simulink model "Deployment_Dispositivo_Gruppo8"  (R2022b)
settings: Solver=FixedStepAuto  StartTime=0.0  StopTime=inf  FixedStep=0.01  RelTol=1e-3  EnableMultiTasking=on
libraries: mbedblockslib x7
settings Model: PacingRate=0.500000  ExtModeTrigDuration=10  Creator=kiraa  LastModifiedBy=kiraa
settings OptimizationCC: EnhancedBackFolding=on  PassReuseOutputArgsAs=Individual arguments  ZeroExternalMemoryAtStartup=off  ZeroInternalMemoryAtStartup=off  MaxStackSize=64  OptimizeBlockOrder=speed  DifferentSizesBufferReuse=on  OptimizationCustomize=off  EfficientTunableParamExpr=on
settings DebuggingCC: ParameterTunabilityLossMsg=error
settings HardwareCC: ProdBitPerPointer=32  ProdBitPerSizeT=32  ProdBitPerPtrDiffT=32  ProdLargestAtomicInteger=Long  ProdLargestAtomicFloat=Double  ProdWordSize=32  ProdLongLongMode=on  ProdHWDeviceType=ARM Compatible->ARM Cortex  UseEmbeddedCoderFeatures=off
settings SFSimCC: MATLABDynamicMemAlloc=off
settings RTWCC: Description=Embedded Coder  SystemTargetFile=ert.tlc  HardwareBoard=STM32 Nucleo F401RE  TLCOptions=-aInlineSetEventsForThisBaseRateFcn=TLC_FALSE -aSuppressMultiTaskScheduler=TLC_FALSE -aRateBasedStepFcn=1  TemplateMakefile=ert_default_tmf  Toolchain=GNU Tools for ARM Embedded Processors
settings CodeAppCC: ForceParamTrailComments=on  IgnoreCustomStorageClasses=off  OperatorAnnotations=on  SimulinkDataObjDesc=on  SFDataObjDesc=on  InsertBlockDesc=on
settings ERTTargetCC: SupportNonInlinedSFcns=on  ExtModeTransport=3  ExtModeStaticAlloc=on  ExtModeStaticAllocSize=2000  ExtModeMexFile=ext_xcp  ExtModeIntrfLevel=Level2 - Open

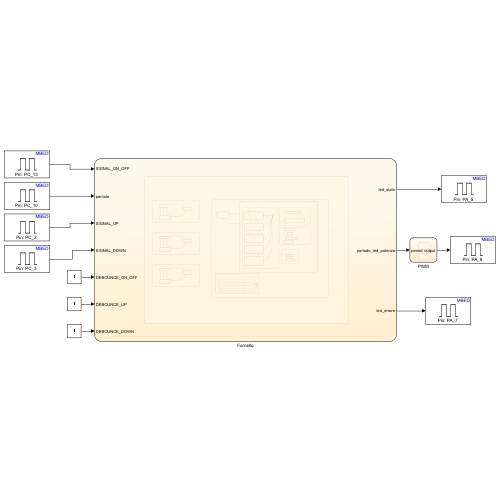
[thumbnail: Simulink's stored preview of the top-level diagram]
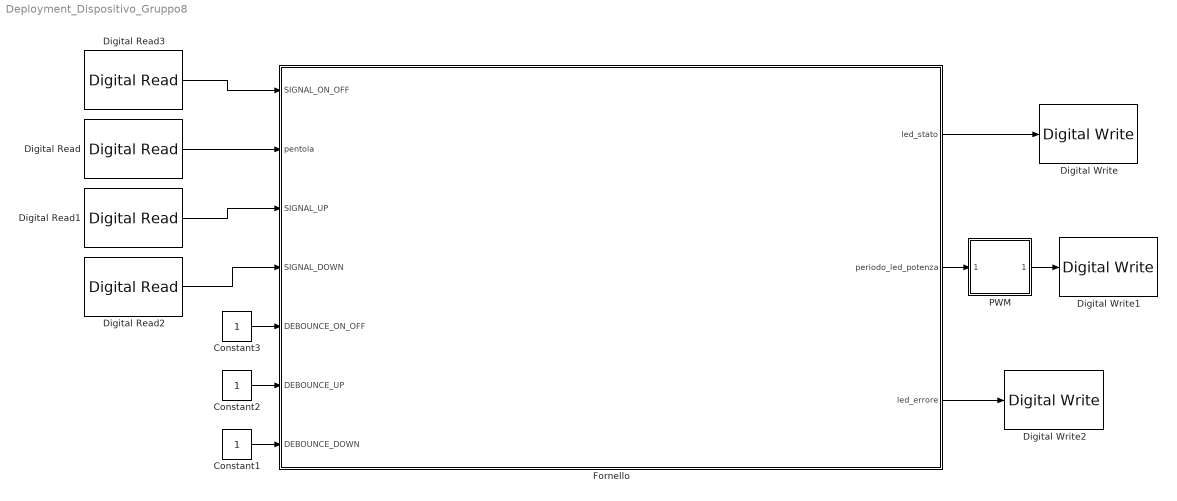
== system Deployment_Dispositivo_Gruppo8 ==
  Constant1 : Constant
  Constant2 : Constant
  Constant3 : Constant
  Digital Read : mbedblockslib/Digital Read  Pin=PC_10  Direction=input  SampleTime=-1
      settings: LibrarySourceBlock=stmnucleorootlib/Common/Digital Read
  Digital Read1 : mbedblockslib/Digital Read  Pin=PC_2  Direction=input  SampleTime=-1
      settings: LibrarySourceBlock=stmnucleorootlib/Common/Digital Read
  Digital Read2 : mbedblockslib/Digital Read  Pin=PC_3  Direction=input  SampleTime=-1
      settings: LibrarySourceBlock=stmnucleorootlib/Common/Digital Read
  Digital Read3 : mbedblockslib/Digital Read  Pin=PC_13  Direction=input  SampleTime=-1
      settings: LibrarySourceBlock=stmnucleorootlib/Common/Digital Read
  Digital Write : mbedblockslib/Digital Write  Pin=PA_5  Direction=output
      settings: LibrarySourceBlock=stmnucleorootlib/Common/Digital Write
  Digital Write1 : mbedblockslib/Digital Write  Pin=PA_6  Direction=output
      settings: LibrarySourceBlock=stmnucleorootlib/Common/Digital Write
  Digital Write2 : mbedblockslib/Digital Write  Pin=PA_7  Direction=output
      settings: LibrarySourceBlock=stmnucleorootlib/Common/Digital Write
  Fornello : Stateflow chart  TreatAsAtomicUnit=on
  PWM : Stateflow chart  TreatAsAtomicUnit=on
  wires:
  Fornello/1(led_stato) -> Digital Write/1
  Fornello/3(led_errore) -> Digital Write2/1
  Fornello/2(periodo_led_potenza) -> PWM/1(period)
  PWM/1(output) -> Digital Write1/1
  Constant1/1 -> Fornello/7(DEBOUNCE_DOWN)
  Constant2/1 -> Fornello/6(DEBOUNCE_UP)
  Constant3/1 -> Fornello/5(DEBOUNCE_ON_OFF)
  Digital Read1/1 -> Fornello/3(SIGNAL_UP)
  Digital Read/1 -> Fornello/2(pentola)
  Digital Read2/1 -> Fornello/4(SIGNAL_DOWN)
  Digital Read3/1 -> Fornello/1(SIGNAL_ON_OFF)

== stateflow chart Deployment_Dispositivo_Gruppo8/Fornello ==
  settings: executeAtInitialization=1
  state DEVICE
    state FORNELLO [parallel]
      settings: executionOrder=1
      state ON
        en: led_stato = true
        state SELECTOR [parallel]
          settings: executionOrder=1
          state SELECTED_0W
            en: selected_power=0;
          state SELECTED_300W
            en: selected_power=300;
          state SELECTED_500W
            en: selected_power=500
          state SELECTED_1000W
            en: selected_power=1000
          state SELECTED_1500W
            en: selected_power=1500
          (default) -> SELECTED_0W
          (junction 32) -> SELECTED_0W
          SELECTED_500W -> (junction 32) [order 1] : disattiva
          SELECTED_1000W -> (junction 32) [order 2] : disattiva
          SELECTED_1500W -> (junction 32) [order 2] : disattiva
          SELECTED_300W -> (junction 32) [order 1] : disattiva
          SELECTED_0W -> SELECTED_300W : LONG_PRESS_UP[pentola == false]
          SELECTED_300W -> SELECTED_0W [order 3] : LONG_PRESS_DOWN[pentola==false]
          SELECTED_500W -> SELECTED_300W [order 2] : LONG_PRESS_DOWN[pentola==false]
          SELECTED_300W -> SELECTED_500W [order 2] : LONG_PRESS_UP[pentola == false]
          SELECTED_1000W -> SELECTED_500W [order 3] : LONG_PRESS_DOWN[pentola==false]
          SELECTED_500W -> SELECTED_1000W [order 3] : LONG_PRESS_UP[pentola == false]
          SELECTED_1500W -> SELECTED_1000W [order 1] : LONG_PRESS_DOWN[pentola == false]
          SELECTED_1000W -> SELECTED_1500W [order 1] : LONG_PRESS_UP[pentola==false]
        state WATCHDOG [parallel]
          settings: executionOrder=2
          state IDLE
          state ERROR
            en: led_errore = true
            on after(10,sec): send(disattiva,SELECTOR); erogaPotenza(0)
            ex: led_errore = false
          (default) -> DEVICE.FORNELLO.ON.WATCHDOG.IDLE
          DEVICE.FORNELLO.ON.WATCHDOG.IDLE -> ERROR : [pentola == true && attivo==true]
          ERROR -> DEVICE.FORNELLO.ON.WATCHDOG.IDLE : [pentola == false || attivo == false]
        state SUPPLIER [parallel]
          settings: executionOrder=3
          state NO_CHANGE_REQUESTED
          state Applying_0_power
            en: erogaPotenza(selected_power)
          state Applying_power
            en: erogaPotenza(selected_power)
          state PENDING_CHANGE
            en: t_debug = 0
          NO_CHANGE_REQUESTED -> PENDING_CHANGE : change_power
          Applying_power -> NO_CHANGE_REQUESTED [order 2]
          Applying_0_power -> NO_CHANGE_REQUESTED
          Applying_power -> Applying_0_power [order 1] : [attivo == false]
          PENDING_CHANGE -> Applying_power : [pentola==false]
        state DELAYED_TRIGGER [parallel]
          settings: executionOrder=4
          state IDLE
          state DELAYING
          (default) -> DEVICE.FORNELLO.ON.DELAYED_TRIGGER.IDLE
          DEVICE.FORNELLO.ON.DELAYED_TRIGGER.IDLE -> DELAYING : change(selected_power)
          DELAYING -> DEVICE.FORNELLO.ON.DELAYED_TRIGGER.IDLE [order 2] : after(5,sec)/{send(change_power, SUPPLIER)}
          DELAYING -> DELAYING [order 1] : change(selected_power)
        (default) -> NO_CHANGE_REQUESTED
      state OFF
        en: led_stato = false; erogaPotenza(0)
      state erogaPotenza(power) [function]
        (default) -> (junction 65) : {power = double(power)}
        (junction 65) -> (junction 68) [order 1] : [power == 0]
        (junction 68) -> (junction 118) : {periodo_led_potenza=0;attivo=false}
        (junction 118) -> (junction 89)
        (junction 65) -> (junction 77) [order 2]
        (junction 77) -> (junction 83) [order 1] : [power == 300]
        (junction 83) -> (junction 120) : {periodo_led_potenza=2;attivo=true}
        (junction 120) -> (junction 89)
        (junction 77) -> (junction 79) [order 2]
        (junction 122) -> (junction 89)
        (junction 119) -> (junction 89)
        (junction 121) -> (junction 89)
        (junction 79) -> (junction 84) [order 1] : [power == 500]
        (junction 84) -> (junction 122) : {periodo_led_potenza=1;attivo=true}
        (junction 79) -> (junction 81) [order 2]
        (junction 81) -> (junction 92) [order 1] : [power == 1000]
        (junction 92) -> (junction 119) : {periodo_led_potenza=0.5;attivo=true}
        (junction 81) -> (junction 95) [order 2]
        (junction 95) -> (junction 99) : [power == 1500]
        (junction 99) -> (junction 121) : {periodo_led_potenza=0.25;attivo=true}
      (default) -> OFF
      OFF -> ON : SHORT_PRESS_ON_OFF
      ON -> OFF : LONG_PRESS_ON_OFF
    state BUTTON_ON_OFF [parallel]
      settings: executionOrder=2
      state HIGH
      state LOW_2
      state LOW
      (default) -> DEVICE.BUTTON_ON_OFF.HIGH
      DEVICE.BUTTON_ON_OFF.LOW_2 -> DEVICE.BUTTON_ON_OFF.HIGH : [SIGNAL_ON_OFF == true]
      DEVICE.BUTTON_ON_OFF.HIGH -> DEVICE.BUTTON_ON_OFF.LOW : [SIGNAL_ON_OFF == false]
      DEVICE.BUTTON_ON_OFF.LOW -> DEVICE.BUTTON_ON_OFF.HIGH [order 2] : before(DEBOUNCE_ON_OFF,sec)[SIGNAL_ON_OFF == true]/{send(SHORT_PRESS_ON_OFF)}
      DEVICE.BUTTON_ON_OFF.LOW -> DEVICE.BUTTON_ON_OFF.HIGH [order 3] : after(DEBOUNCE_ON_OFF,sec)[SIGNAL_ON_OFF == true]/{send(LONG_PRESS_ON_OFF)}
      DEVICE.BUTTON_ON_OFF.LOW -> DEVICE.BUTTON_ON_OFF.LOW_2 [order 1] : after(DEBOUNCE_ON_OFF,sec)[SIGNAL_ON_OFF == false]/{send(LONG_PRESS_ON_OFF)}
    state BUTTON_UP [parallel]
      settings: executionOrder=3
      state HIGH
      state LOW_2
      state LOW
      (default) -> DEVICE.BUTTON_UP.HIGH
      DEVICE.BUTTON_UP.LOW_2 -> DEVICE.BUTTON_UP.HIGH : [SIGNAL_UP == true]
      DEVICE.BUTTON_UP.HIGH -> DEVICE.BUTTON_UP.LOW : [SIGNAL_UP == false]
      DEVICE.BUTTON_UP.LOW -> DEVICE.BUTTON_UP.HIGH [order 2] : before(DEBOUNCE_UP,sec)[SIGNAL_UP == true]/{send(SHORT_PRESS_UP)}
      DEVICE.BUTTON_UP.LOW -> DEVICE.BUTTON_UP.HIGH [order 3] : after(DEBOUNCE_UP,sec)[SIGNAL_UP == true]/{send(LONG_PRESS_UP)}
      DEVICE.BUTTON_UP.LOW -> DEVICE.BUTTON_UP.LOW_2 [order 1] : after(DEBOUNCE_UP,sec)[SIGNAL_UP == false]/{send(LONG_PRESS_UP)}
    state BUTTON_DOWN [parallel]
      settings: executionOrder=4
      state HIGH
      state LOW_2
      state LOW
      (default) -> DEVICE.BUTTON_DOWN.HIGH
      DEVICE.BUTTON_DOWN.LOW_2 -> DEVICE.BUTTON_DOWN.HIGH : [SIGNAL_DOWN == true]
      DEVICE.BUTTON_DOWN.HIGH -> DEVICE.BUTTON_DOWN.LOW : [SIGNAL_DOWN == false]
      DEVICE.BUTTON_DOWN.LOW -> DEVICE.BUTTON_DOWN.HIGH [order 2] : before(DEBOUNCE_DOWN,sec)[SIGNAL_DOWN == true]/{send(SHORT_PRESS_DOWN)}
      DEVICE.BUTTON_DOWN.LOW -> DEVICE.BUTTON_DOWN.HIGH [order 3] : after(DEBOUNCE_DOWN,sec)[SIGNAL_DOWN == true]/{send(LONG_PRESS_DOWN)}
      DEVICE.BUTTON_DOWN.LOW -> DEVICE.BUTTON_DOWN.LOW_2 [order 1] : after(DEBOUNCE_DOWN,sec)[SIGNAL_DOWN == false]/{send(LONG_PRESS_DOWN)}
  (default) -> DEVICE
  data: power function_input double size=1; SIGNAL_ON_OFF input; attivo local boolean size=1 =false; led_stato output boolean size=1 =false; periodo_led_potenza output double size=1 =0; led_errore output boolean size=1 =false; pentola input boolean size=1; SIGNAL_UP input; SIGNAL_DOWN input; DEBOUNCE_ON_OFF input double; DEBOUNCE_UP input double; selected_power local double size=1 =0; t_debug local double =1; last_down local; last_up local; DEBOUNCE_DOWN input double; last_on_off local; debug local; flag local =0; last_value local
  events: disattiva local FUNCTION_CALL_EVENT; change_power local FUNCTION_CALL_EVENT; LONG_PRESS_DOWN local FUNCTION_CALL_EVENT; LONG_PRESS_UP local FUNCTION_CALL_EVENT; SHORT_PRESS_DOWN local FUNCTION_CALL_EVENT; SHORT_PRESS_UP local FUNCTION_CALL_EVENT; LONG_PRESS_ON_OFF local FUNCTION_CALL_EVENT; SHORT_PRESS_ON_OFF local FUNCTION_CALL_EVENT

== stateflow chart Deployment_Dispositivo_Gruppo8/PWM ==
  state Off
    en: output = false
  state On
    en: output = true
  (default) -> Off
  Off -> On : after(period,sec)[period ~= 0]
  On -> Off : after(period,sec)
  data: output output boolean size=1 =false; period input double size=1
